simulink model "F16_Model_"  (R2025b)
settings: Solver=VariableStepAuto  StartTime=0.0  StopTime=100  RelTol=1e-3
values from neighbouring files (symbols this model uses):
  aero_data =     [aero_data.mat]
  b = 9.144    [initialization.m]
  c_bar = 3.45    [initialization.m]
  g = 9.81    [initialization.m]
  initial_pow = 50    [controlInputs.m]
  mass = 9295.4128    [initialization.m]
  S = 27.87    [initialization.m]
  u1 = 0    [controlInputs.m]
  u2 = 0    [controlInputs.m]
  u3 = -2    [controlInputs.m]
  u4 = 0    [controlInputs.m]
  u5 = 0    [controlInputs.m]
  u6 = 0.6    [controlInputs.m]
  xcg = 0.3*c_bar    (= 1.035)    [initialization.m]
  xcgr = 0.35*c_bar    (= 1.2075)    [initialization.m]
libraries: simulink_extras x9, aerolibfltsims x2, aerolibobsolete x1
(part 2 of 2)

== system F16_Model_/AeroForcesMoments/Aerodynamics/Cn/Leading Edge Flap Adjustment ==
  alpha : Inport
  beta : Inport  Port=2
  del_lef : Inport  Port=3
  Cn_del_h_0 : Lookup_n-D  BreakpointsForDimension1=[-20, -15, -10, -5, 0, 5, 10, 15, 20, 25, 30, 35, 40, 45, 50, 55, 60, 70, 80, 90];  BreakpointsForDimension2=[-30, -25, -20, -15, -10, -8, -6, -4, -2, 0, 2, 4, 6, 8, 10, 15, 20, 25, 30];  Table=aero_data.Cn_del_h_0  InternalRulePriority=Speed  RndMeth=Simplest
      settings: InputPortMap=u0,u1
  Cn_lef : Lookup_n-D  BreakpointsForDimension1=[-20, -15, -10, -5, 0, 5, 10, 15, 20, 25, 30, 35, 40, 45];  BreakpointsForDimension2=[-30, -25, -20, -15, -10, -8, -6, -4, -2, 0, 2, 4, 6, 8, 10, 15, 20, 25, 30];  Table=aero_data.Cn_lef  InternalRulePriority=Speed  RndMeth=Simplest
      settings: InputPortMap=u0,u1
  Constant : Constant
  Multiply : Gain  Gain=0.04
  Product : Product
  Subtract : Sum  Inputs=+-
  Subtract1 : Sum  Inputs=+-
  Out1 : Outport
  wires:
  alpha/1 -> Cn_del_h_0/1, Cn_lef/1
  Cn_lef/1 -> Subtract1/1
  Cn_del_h_0/1 -> Subtract1/2
  beta/1 -> Cn_del_h_0/2, Cn_lef/2
  del_lef/1 -> Multiply/1
  Constant/1 -> Subtract/1
  Multiply/1 -> Subtract/2
  Subtract/1 -> Product/2
  Subtract1/1 -> Product/1
  Product/1 -> Out1/1

== system F16_Model_/AeroForcesMoments/Aerodynamics/Cn/Roll Rate Damping ==
  alpha : Inport
  del_lef : Inport  Port=2
  p : Inport  Port=3
  Add : Sum
  Cn_p : Lookup_n-D  NumberOfTableDimensions=1  BreakpointsForDimension1=[-20, -15, -10, -5, 0, 5, 10, 15, 20, 25, 30, 35, 40, 45, 50, 55, 60, 70, 80, 90];  Table=aero_data.Cnp  InternalRulePriority=Speed  RndMeth=Simplest
  Constant : Constant
  Constant1 : Constant  Value=25
  Divide : Product  Inputs=*/
  Product : Product
  Product1 : Product
  Subtract : Sum  Inputs=+-
  del_Cn_p_lef : Lookup_n-D  NumberOfTableDimensions=1  BreakpointsForDimension1=[-20, -15, -10, -5, 0, 5, 10, 15, 20, 25, 30, 35, 40, 45];  Table=aero_data.del_Cn_p_lef  InternalRulePriority=Speed  RndMeth=Simplest
  Out1 : Outport
  wires:
  alpha/1 -> del_Cn_p_lef/1, Cn_p/1
  del_Cn_p_lef/1 -> Product/1  "del_Cn_p_lef"
  Cn_p/1 -> Add/1
  del_lef/1 -> Divide/1
  Constant1/1 -> Divide/2
  Constant/1 -> Subtract/1
  Divide/1 -> Subtract/2
  Subtract/1 -> Product/2  "1 - del_lef/25"
  Product/1 -> Add/2
  Add/1 -> Product1/1
  p/1 -> Product1/2
  Product1/1 -> Out1/1

== system F16_Model_/AeroForcesMoments/Aerodynamics/Cn/Rudder Adjustment ==
  alpha : Inport
  beta : Inport  Port=2
  del_r : Inport  Port=3
  Cn_del_h_0 : Lookup_n-D  BreakpointsForDimension1=[-20, -15, -10, -5, 0, 5, 10, 15, 20, 25, 30, 35, 40, 45, 50, 55, 60, 70, 80, 90];  BreakpointsForDimension2=[-30, -25, -20, -15, -10, -8, -6, -4, -2, 0, 2, 4, 6, 8, 10, 15, 20, 25, 30];  Table=aero_data.Cn_del_h_0  InternalRulePriority=Speed  RndMeth=Simplest
      settings: InputPortMap=u0,u1
  Cn_del_r_30 : Lookup_n-D  BreakpointsForDimension1=[-20, -15, -10, -5, 0, 5, 10, 15, 20, 25, 30, 35, 40, 45, 50, 55, 60, 70, 80, 90];  BreakpointsForDimension2=[-30, -25, -20, -15, -10, -8, -6, -4, -2, 0, 2, 4, 6, 8, 10, 15, 20, 25, 30];  Table=aero_data.Cn_del_r_30  InternalRulePriority=Speed  RndMeth=Simplest
      settings: InputPortMap=u0,u1
  Multiply : Gain  Gain=1/30
  Product : Product
  Subtract : Sum  Inputs=+-
  Out1 : Outport
  wires:
  beta/1 -> Cn_del_h_0/2, Cn_del_r_30/2
  Cn_del_h_0/1 -> Subtract/2
  Cn_del_r_30/1 -> Subtract/1
  alpha/1 -> Cn_del_h_0/1, Cn_del_r_30/1
  del_r/1 -> Multiply/1
  Subtract/1 -> Product/1
  Multiply/1 -> Product/2
  Product/1 -> Out1/1

== system F16_Model_/AeroForcesMoments/Aerodynamics/Cn/Yaw Rate Damping ==
  alpha : Inport
  del_lef : Inport  Port=2
  r : Inport  Port=3
  Add : Sum
  Cn_r : Lookup_n-D  NumberOfTableDimensions=1  BreakpointsForDimension1=[-20, -15, -10, -5, 0, 5, 10, 15, 20, 25, 30, 35, 40, 45, 50, 55, 60, 70, 80, 90];  Table=aero_data.Cnr  InternalRulePriority=Speed  RndMeth=Simplest
  Constant : Constant
  Constant1 : Constant  Value=25
  Divide : Product  Inputs=*/
  Product : Product
  Product1 : Product
  Subtract : Sum  Inputs=+-
  del_Cl_r_lef : Lookup_n-D  NumberOfTableDimensions=1  BreakpointsForDimension1=[-20, -15, -10, -5, 0, 5, 10, 15, 20, 25, 30, 35, 40, 45];  Table=aero_data.del_Cn_r_lef  InternalRulePriority=Speed  RndMeth=Simplest
  Out1 : Outport
  wires:
  Cn_r/1 -> Add/1
  alpha/1 -> del_Cl_r_lef/1, Cn_r/1
  del_Cl_r_lef/1 -> Product/1
  del_lef/1 -> Divide/1
  Divide/1 -> Subtract/2
  Subtract/1 -> Product/2  "1 - del_lef/25"
  Constant/1 -> Subtract/1
  Constant1/1 -> Divide/2
  Product/1 -> Add/2
  Add/1 -> Product1/1
  r/1 -> Product1/2
  Product1/1 -> Out1/1

== system F16_Model_/AeroForcesMoments/Aerodynamics/Cx/Leading Edge flap Adjustment ==
  alpha : Inport
  beta : Inport  Port=2
  del_lef : Inport  Port=3
  Constant : Constant
  Constant1 : Constant  Value=25
  Cx_del_h_0 : Lookup_n-D  BreakpointsForDimension1=[-20, -15, -10, -5, 0, 5, 10, 15, 20, 25, 30, 35, 40, 45, 50, 55, 60, 70, 80, 90];  BreakpointsForDimension2=[-30, -25, -20, -15, -10, -8, -6, -4, -2, 0, 2, 4, 6, 8, 10, 15, 20, 25, 30];  Table=aero_data.Cx_del_h_0  InternalRulePriority=Speed  RndMeth=Simplest
      settings: InputPortMap=u0,u1
  Cx_lef : Lookup_n-D  BreakpointsForDimension1=[-20, -15, -10, -5, 0, 5, 10, 15, 20, 25, 30, 35, 40, 45];  BreakpointsForDimension2=[-30, -25, -20, -15, -10, -8, -6, -4, -2, 0, 2, 4, 6, 8, 10, 15, 20, 25, 30];  Table=aero_data.Cx_lef  InternalRulePriority=Speed  RndMeth=Simplest
      settings: InputPortMap=u0,u1
  Divide : Product  Inputs=*/
  Product : Product
  Subtract : Sum  Inputs=+-
  Subtract1 : Sum  Inputs=+-
  Out1 : Outport
  wires:
  alpha/1 -> Cx_lef/1, Cx_del_h_0/1
  Subtract/1 -> Product/1
  Cx_del_h_0/1 -> Subtract/2  "Cx_del_h_10"
  Product/1 -> Out1/1
  Cx_lef/1 -> Subtract/1  "Cx_lef"
  beta/1 -> Cx_lef/2, Cx_del_h_0/2
  del_lef/1 -> Divide/1
  Constant1/1 -> Divide/2
  Constant/1 -> Subtract1/1
  Divide/1 -> Subtract1/2
  Subtract1/1 -> Product/2

== system F16_Model_/AeroForcesMoments/Aerodynamics/Cx/Pitching Rate Damping ==
  note: (c_bar*q)/(2*V)
  alpha : Inport
  q : Inport  Port=2
  V : Inport  Port=3
  del_lef : Inport  Port=4
  Add : Sum
  Constant : Constant  Value=c_bar
  Constant1 : Constant  Value=2
  Constant2 : Constant
  Constant3 : Constant  Value=25
  Cxq : Lookup_n-D  NumberOfTableDimensions=1  BreakpointsForDimension1=[-20, -15, -10, -5, 0, 5, 10, 15, 20, 25, 30, 35, 40, 45, 50, 55, 60, 70, 80, 90];  Table=aero_data.Cxq  InternalRulePriority=Speed  RndMeth=Simplest
  Divide : Product  Inputs=*/
  Divide1 : Product  Inputs=*/
  Product{,1..3} (4 alike) : Product
  Subtract1 : Sum  Inputs=+-
  del_Cxq_lef : Lookup_n-D  NumberOfTableDimensions=1  BreakpointsForDimension1=[-20, -15, -10, -5, 0, 5, 10, 15, 20, 25, 30, 35, 40, 45];  Table=aero_data.del_Cxq_lef  InternalRulePriority=Speed  RndMeth=Simplest
  Out1 : Outport
  wires:
  Add/1 -> Product2/1
  Product3/1 -> Add/2
  Cxq/1 -> Add/1  "Cxq"
  del_Cxq_lef/1 -> Product3/1  "del_Cxq_lef"
  Product2/1 -> Out1/1
  alpha/1 -> Cxq/1, del_Cxq_lef/1
  q/1 -> Product/1
  Constant/1 -> Product/2
  Product/1 -> Divide/1
  Constant1/1 -> Product1/1
  V/1 -> Product1/2
  Product1/1 -> Divide/2
  Divide/1 -> Product2/2
  Constant2/1 -> Subtract1/1
  Divide1/1 -> Subtract1/2
  Subtract1/1 -> Product3/2
  del_lef/1 -> Divide1/1
  Constant3/1 -> Divide1/2

== system F16_Model_/AeroForcesMoments/Aerodynamics/Cx/Speed Brake ==
  alpha : Inport
  del_sb : Inport  Port=2
  Constant : Constant  Value=60
  Divide : Product  Inputs=*/
  Product : Product
  delCx_sb : Lookup_n-D  NumberOfTableDimensions=1  BreakpointsForDimension1=[-20, -15, -10, -5, 0, 5, 10, 15, 20, 25, 30, 35, 40, 45, 50, 55, 60, 70, 80, 90];  Table=aero_data.del_Cx_sb  InternalRulePriority=Speed  RndMeth=Simplest
  Out1 : Outport
  wires:
  delCx_sb/1 -> Product/1  "del_Cx_sb"
  Product/1 -> Out1/1
  alpha/1 -> delCx_sb/1
  del_sb/1 -> Divide/1
  Constant/1 -> Divide/2
  Divide/1 -> Product/2

== system F16_Model_/AeroForcesMoments/Aerodynamics/Cz/Leading Edge Flap Adjustment ==
  alpha : Inport
  beta : Inport  Port=2
  del_lef : Inport  Port=3
  Constant : Constant
  Constant1 : Constant  Value=25
  Cz_del_h_0 : Lookup_n-D  BreakpointsForDimension1=[-20, -15, -10, -5, 0, 5, 10, 15, 20, 25, 30, 35, 40, 45, 50, 55, 60, 70, 80, 90];  BreakpointsForDimension2=[-30, -25, -20, -15, -10, -8, -6, -4, -2, 0, 2, 4, 6, 8, 10, 15, 20, 25, 30];  Table=aero_data.Cz_del_h_0  InternalRulePriority=Speed  RndMeth=Simplest
      settings: InputPortMap=u0,u1
  Cz_lef : Lookup_n-D  BreakpointsForDimension1=[-20, -15, -10, -5, 0, 5, 10, 15, 20, 25, 30, 35, 40, 45];  BreakpointsForDimension2=[-30, -25, -20, -15, -10, -8, -6, -4, -2, 0, 2, 4, 6, 8, 10, 15, 20, 25, 30];  Table=aero_data.Cz_lef  InternalRulePriority=Speed  RndMeth=Simplest
      settings: InputPortMap=u0,u1
  Divide : Product  Inputs=*/
  Product : Product
  Subtract : Sum  Inputs=+-
  Subtract1 : Sum  Inputs=+-
  Out1 : Outport
  wires:
  alpha/1 -> Cz_lef/1, Cz_del_h_0/1
  Subtract/1 -> Product/1
  Cz_del_h_0/1 -> Subtract/2  "Cx_del_h_0"
  Product/1 -> Out1/1
  Cz_lef/1 -> Subtract/1  "Cz_lef"
  beta/1 -> Cz_lef/2, Cz_del_h_0/2
  del_lef/1 -> Divide/1
  Constant1/1 -> Divide/2
  Constant/1 -> Subtract1/1
  Divide/1 -> Subtract1/2
  Subtract1/1 -> Product/2

== system F16_Model_/AeroForcesMoments/Aerodynamics/Cz/Pitching Rate Damping ==
  note: (c_bar*q)/(2*V)
  alpha : Inport
  q : Inport  Port=2
  V : Inport  Port=3
  del_lef : Inport  Port=4
  Add : Sum
  Constant : Constant  Value=c_bar
  Constant1 : Constant  Value=2
  Constant2 : Constant
  Constant3 : Constant  Value=25
  Czq : Lookup_n-D  NumberOfTableDimensions=1  BreakpointsForDimension1=[-20, -15, -10, -5, 0, 5, 10, 15, 20, 25, 30, 35, 40, 45, 50, 55, 60, 70, 80, 90];  Table=aero_data.Czq  InternalRulePriority=Speed  RndMeth=Simplest
  Divide : Product  Inputs=*/
  Divide1 : Product  Inputs=*/
  Product{,1..3} (4 alike) : Product
  Subtract1 : Sum  Inputs=+-
  delCzq_lef : Lookup_n-D  NumberOfTableDimensions=1  BreakpointsForDimension1=[-20, -15, -10, -5, 0, 5, 10, 15, 20, 25, 30, 35, 40, 45];  Table=aero_data.delCzq_lef  InternalRulePriority=Speed  RndMeth=Simplest
  Out1 : Outport
  wires:
  Add/1 -> Product2/1
  Product3/1 -> Add/2
  Czq/1 -> Add/1  "Czq"
  delCzq_lef/1 -> Product3/1  "delCzq_lef"
  Product2/1 -> Out1/1
  alpha/1 -> Czq/1, delCzq_lef/1
  q/1 -> Product/1
  Constant/1 -> Product/2
  Product/1 -> Divide/1
  Constant1/1 -> Product1/1
  V/1 -> Product1/2
  Product1/1 -> Divide/2
  Divide/1 -> Product2/2
  Constant2/1 -> Subtract1/1
  Divide1/1 -> Subtract1/2
  Subtract1/1 -> Product3/2
  del_lef/1 -> Divide1/1
  Constant3/1 -> Divide1/2

== system F16_Model_/AeroForcesMoments/Aerodynamics/Cz/Speed Brake ==
  alpha : Inport
  del_sb : Inport  Port=2
  Constant : Constant  Value=60
  Divide : Product  Inputs=*/
  Product : Product
  delCz_sb : Lookup_n-D  NumberOfTableDimensions=1  BreakpointsForDimension1=[-20, -15, -10, -5, 0, 5, 10, 15, 20, 25, 30, 35, 40, 45, 50, 55, 60, 70, 80, 90];  Table=aero_data.delCz_sb  InternalRulePriority=Speed  RndMeth=Simplest
  Out1 : Outport
  wires:
  delCz_sb/1 -> Product/1  "delCz_sb"
  Product/1 -> Out1/1
  alpha/1 -> delCz_sb/1
  del_sb/1 -> Divide/1
  Constant/1 -> Divide/2
  Divide/1 -> Product/2

== system F16_Model_/AeroForcesMoments/Aerodynamics/C_y/Aileron Adjustment/del_Cy_del_a_20*(1-del_lef//25) ==
  alpha : Inport
  beta : Inport  Port=2
  del_lef : Inport  Port=3
  Constant1 : Constant
  Constant2 : Constant  Value=25
  Cy_del_a_20_lef : Lookup_n-D  BreakpointsForDimension1=[-20, -15, -10, -5, 0, 5, 10, 15, 20, 25, 30, 35, 40, 45];  BreakpointsForDimension2=[-30, -25, -20, -15, -10, -8, -6, -4, -2, 0, 2, 4, 6, 8, 10, 15, 20, 25, 30];  Table=aero_data.Cy_del_a_20_lef  InternalRulePriority=Speed  RndMeth=Simplest
      settings: InputPortMap=u0,u1
  Cy_lef : Lookup_n-D  BreakpointsForDimension1=[-20, -15, -10, -5, 0, 5, 10, 15, 20, 25, 30, 35, 40, 45];  BreakpointsForDimension2=[-30, -25, -20, -15, -10, -8, -6, -4, -2, 0, 2, 4, 6, 8, 10, 15, 20, 25, 30];  Table=aero_data.Cy_lef  InternalRulePriority=Speed  RndMeth=Simplest
      settings: InputPortMap=u0,u1
  Divide1 : Product  Inputs=*/
  Product2 : Product
  Subtract2 : Sum  Inputs=+-
  Subtract3 : Sum  Inputs=+-
  Out1 : Outport
  wires:
  Constant1/1 -> Subtract3/1
  alpha/1 -> Cy_lef/1, Cy_del_a_20_lef/1
  beta/1 -> Cy_lef/2, Cy_del_a_20_lef/2
  Subtract3/1 -> Product2/2  "1 - del_lef/25"
  Subtract2/1 -> Product2/1
  Cy_lef/1 -> Subtract2/2  "Cy_lef"
  Constant2/1 -> Divide1/2
  Product2/1 -> Out1/1
  del_lef/1 -> Divide1/1
  Divide1/1 -> Subtract3/2
  Cy_del_a_20_lef/1 -> Subtract2/1  "Cy_del_a_20_lef"

== system F16_Model_/AeroForcesMoments/Aerodynamics/C_y/Flap Adjustment/1-del_lef//25 ==
  del_lef1 : Inport
  Constant1 : Constant
  Constant2 : Constant  Value=25
  Divide1 : Product  Inputs=*/
  Subtract3 : Sum  Inputs=+-
  1 - del_lef/25 : Outport
  wires:
  Constant1/1 -> Subtract3/1
  Subtract3/1 -> 1 - del_lef/25/1  "1 - del_lef/25"
  Divide1/1 -> Subtract3/2
  del_lef1/1 -> Divide1/1
  Constant2/1 -> Divide1/2

== matlab function F16_Model_/AeroForcesMoments/MATLAB Function ==
  data: F_stability input; F_body output; alpha input
function F_body = fcn(F_stability, alpha)
C_bs = [cos(alpha) 0 -sin(alpha);
        0 1 0;
        sin(alpha) 0 cos(alpha)];
F_body = C_bs*F_stability;

end

== matlab function F16_Model_/Engine/Thrust_ ==
  data: POW input; THRUST output; ALT input; MACH input
function THRUST = THRUST(POW, ALT, MACH)
Mach = [0.2, 0.4, 0.6, 0.8, 1.0];
altitudes = [0, 3048, 6096, 9144, 12192, 15240];

T_idle = [
    2824, 1890, 3069, 4492, 5916, 7562;
    267, 111, 1535, 3358, 5026, 6783;
    -4537, -3158, -1334, 1557, 4048, 6049;
    -12010, -8451, -5782, -1099, 2669, 4893;
    -16013, -6227, -2647, -1521, -890, 3114;
    ];

T_mil = [
    56401, 40699, 28080, 17970, 10987, 6227;
    56089, 41420, 29401, 19082, 11565, 6939;
    56223, 43764, 31536, 20728, 12632, 7384;
    55111, 45263, 34472, 23663, 14456, 8585;
    51953, 43804, 35806, 27133, 16902, 10275;
    ];

T_max = [
    95276, 69834, 49929, 32573, 19727, 11565;
    100970, 74993, 54488, 36269, 22240, 12610;
    107820, 84112, 61204, 41300, 25354, 14300;
    115959, 93742, 71057, 49440, 30513, 17570;
    128485, 103723, 81398, 59977, 38440, 22494;
    ];

% Clamp inputs to data range
ALT = max(0, min(ALT, 15240));
MACH = max(0.2, min(MACH, 1.0));
POW = max(0, min(POW, 100));

% Perform 2D interpolation
T_idle_interp = interp2(altitudes, Mach, T_idle, ALT, MACH, 'linear', 0);
T_mil_interp = interp2(altitudes, Mach, T_mil, ALT, MACH, 'linear', 0);
T_max_interp = interp2(altitudes, Mach, T_max, ALT, MACH, 'linear', 0);

% Handle NaN from interpolation (e.g., edge cases)
T_idle_interp = max(T_idle_interp, 0); % Avoid negative thrust
T_mil_interp = max(T_mil_interp, 0);
T_max_interp = max(T_max_interp, 0);

% Calculate thrust based on power
if POW < 50
    THRUST = T_idle_interp + (T_mil_interp - T_idle_interp) * (POW * 0.02);
else
    THRUST = T_mil_interp + (T_max_interp - T_mil_interp) * ((POW - 50) * 0.02);
end

if isinf(THRUST) || isnan(THRUST)
    THRUST = 0;
    
end

== matlab function F16_Model_/Engine/TGEAR ==
  data: THTL input; TGEAR output
% TGEAR: Computes the power command (TGEAR) based on the throttle setting (THTL).
% Purpose: Translates the pilot's throttle input (a normalized value between 0 and 1) 
%          into a power command that the engine control system can use. This function 
%          models the nonlinear relationship between throttle position and engine power 
%          demand, derived from empirical data for the F-16 engine.
% Why Used: It provides a realistic interface between the pilot's control input and 
%           the engine's power dynamics, ensuring accurate power commands (P1) for 
%           subsequent dynamic calculations. The piecewise linear mapping accounts 
%           for different engine operating regimes (e.g., low power vs. high power).
% Input: THTL - Throttle setting (normalized, 0 to 1)
% Output: TGEAR - Power command value (in arbitrary units, e.g., % or scaled power)


function TGEAR = TGEAR(THTL)
% Clamp THTL to [0, 1]
THTL = max(0, min(THTL, 1));

if THTL <= 0.77
    TGEAR = 64.94 * THTL;
else
    TGEAR = 217.38 * THTL - 117.38;
end
end

== matlab function F16_Model_/Engine/PDOT ==
  data: P3 input; PDOT output; P1 input
% PDOT: Computes the rate of change of actual power (PDOT) based on the power command (P1) 
%       and current actual power (P3).
% Purpose: Models the dynamic response of the engine by calculating how quickly the actual 
%          power (P3) should adjust toward the commanded power (P1). This introduces a 
%          first-order lag to simulate real engine behavior, preventing abrupt power changes.
% Why Used: It ensures a smooth transition of engine power in response to throttle inputs, 
%           which is critical for flight stability, especially in a fighter aircraft like 
%           the F-16 operating near stall/post-stall conditions. The threshold (50.0) 
%           differentiates low-power and high-power regimes with different time constants.
% Input: P3 - Actual power (in arbitrary units, e.g., % or kW)
%        P1 - Power command (from TGEAR, same units as P3)
% Output: PDOT - Rate of change of power (units: power/time, e.g., %/s or kW/s)




function PDOT = PDOT(P3, P1)
P1 = max(0, min(P1, 100));
P3 = max(0, min(P3, 100));

if P1 >= 50
    if P3 >= 50
        TF = 5.0;
        P2 = P1;
    else
        P2 = 60;
        TF = TAU(P2 - P3);
    end
else
    if P3 >= 50
        TF = 5.0;
        P2 = 40;
    else
        P2 = P1;
        TF = TAU(P2 - P3);
    end
end
PDOT = TF * (P2 - P3);
PDOT = max(PDOT, -P3); % Prevent P3 from going negative
end


function TAU = TAU(DP)
DP = max(0, min(DP, 100));
if DP <= 25
    TAU = 1.0;
elseif DP >= 50
    TAU = 0.1;
else
    % Linear interpolation between (25, 1.0) and (50, 0.1)
    TAU = 1.0 - (DP - 25) * (1.0 - 0.1) / (50 - 25);
end
end
